simulink model "Week2"  (R2023b)
settings: Solver=ode1  StartTime=0.0  StopTime=25  FixedStep=0.1  RelTol=1e-3
values from neighbouring files (symbols this model uses):
  A = A_a(2)    [Project1.m]    (also in Project1_and_graphing.m; Project1_and_graphing_plz_check.m; Project1_week1.m = 4; Project1_week2.m = [0, 100])
  b = b_a(q)    [Project1.m]    (also in Project1_and_graphing.m; Project1_and_graphing_plz_check.m; Project1_week1.m = 1; Project1_week2.m = [10, 0.1])
  J = J_a(r)    [Project1.m]    (also in Project1_and_graphing.m; Project1_and_graphing_plz_check.m; Project1_week1.m = 1; Project1_week2.m = [100, 0.01])
  w_0 = 1.0    (= 1)    [Project1_week1.m]    (also in Project1_week2.m = [10, 0])
settings Model: Creator=vince  LastModifiedBy=vince

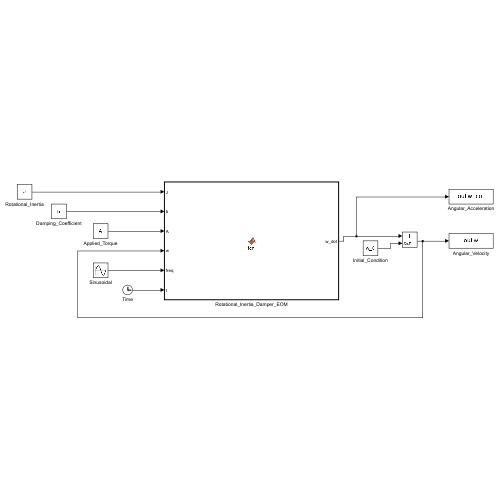
[thumbnail: Simulink's stored preview of the top-level diagram]
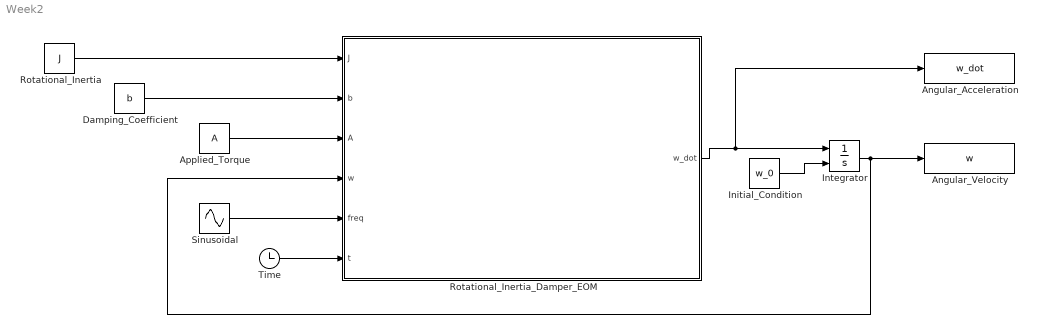
== system Week2 ==
  Angular_Acceleration : ToWorkspace  VariableName=w_dot  SaveFormat=Timeseries  SampleTime=-1
  Angular_Velocity : ToWorkspace  VariableName=w  SaveFormat=Timeseries  SampleTime=-1
  Applied_Torque : Constant  Value=A
  Damping_Coefficient : Constant  Value=b
  Initial_Condition : Constant  Value=w_0
  Integrator : Integrator  InitialConditionSource=external
  Rotational_Inertia : Constant  Value=J
  Rotational_Inertia_Damper_EOM : MATLAB Function  TreatAsAtomicUnit=on
  Sinusoidal : Sin  Amplitude=100  Frequency=0.1  SampleTime=0
  Time : Clock
  wires:
  Rotational_Inertia/1 -> Rotational_Inertia_Damper_EOM/1(J)
  Damping_Coefficient/1 -> Rotational_Inertia_Damper_EOM/2(b)
  Applied_Torque/1 -> Rotational_Inertia_Damper_EOM/3(A)
  Rotational_Inertia_Damper_EOM/1(w_dot) -> Angular_Acceleration/1, Integrator/1
  Initial_Condition/1 -> Integrator/2
  Integrator/1 -> Rotational_Inertia_Damper_EOM/4(w), Angular_Velocity/1
  Time/1 -> Rotational_Inertia_Damper_EOM/6(t)
  Sinusoidal/1 -> Rotational_Inertia_Damper_EOM/5(freq)

== matlab function Week2/Rotational_Inertia_Damper_EOM ==
  data: J input; w_dot output; b input; A input; w input; freq input; t input
function w_dot = fcn(J, b, A, w, freq, t)
    tau_damped = b*w;
    tau = A*sin(freq*t);
    w_dot = (1/J)*(A - b*w);
end
